simulink model "gen_plant"  (R2024b)
settings: Solver=VariableStepAuto  StartTime=0.0  StopTime=10.0  RelTol=1e-3
values from neighbouring files (symbols this model uses):
  Ga = 0.095    [lab09_01_01.m]
  Gf = 1    [lab09_01_01.m]
  Gs = 1    [lab09_01_01.m]
libraries: cstblocks x3
settings Model: Creator=adrian  LastModifiedBy=adrian

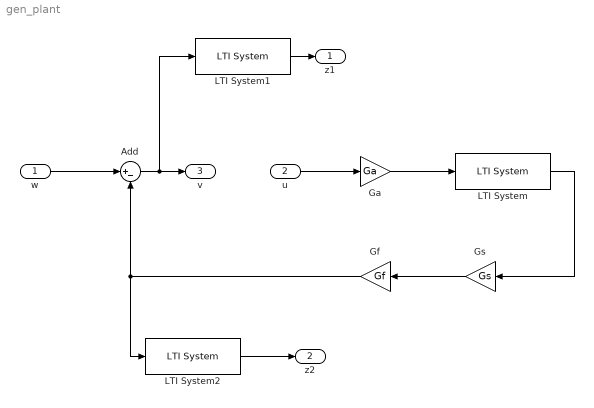
== system gen_plant ==
  w : Inport
  u : Inport  Port=2
  Add : Sum  Inputs=|+-
  Ga : Gain  Gain=Ga
  Gf : Gain  Gain=Gf
  Gs : Gain  Gain=Gs
  LTI System : cstblocks/LTI System  sys=Gpn  IC=[]  PadeOrder=0
  LTI System1 : cstblocks/LTI System  sys=W1mod  IC=[]  PadeOrder=0
  LTI System2 : cstblocks/LTI System  sys=W2mod  IC=[]  PadeOrder=0
  z1 : Outport
  z2 : Outport  Port=2
  v : Outport  Port=3
  wires:
  Ga/1 -> LTI System/1
  LTI System/1 -> Gs/1
  Gs/1 -> Gf/1
  Gf/1 -> Add/2, LTI System2/1
  w/1 -> Add/1
  Add/1 -> LTI System1/1, v/1
  u/1 -> Ga/1
  LTI System1/1 -> z1/1
  LTI System2/1 -> z2/1
